simulink model "CCf"  (Simulink 7.5)
settings: Solver=ode45  StartTime=0.0  StopTime=60  RelTol=1e-3
StartFcn:
  | faHPGR=[0.0239 0.4001 0.2089 0.1090 0.0549 0.0441 0.0542 0.0374 0.0159 0.0085 0.0088 0.0085 0.0258]
settings Model: Creator=Fer  LastModifiedBy=Fer

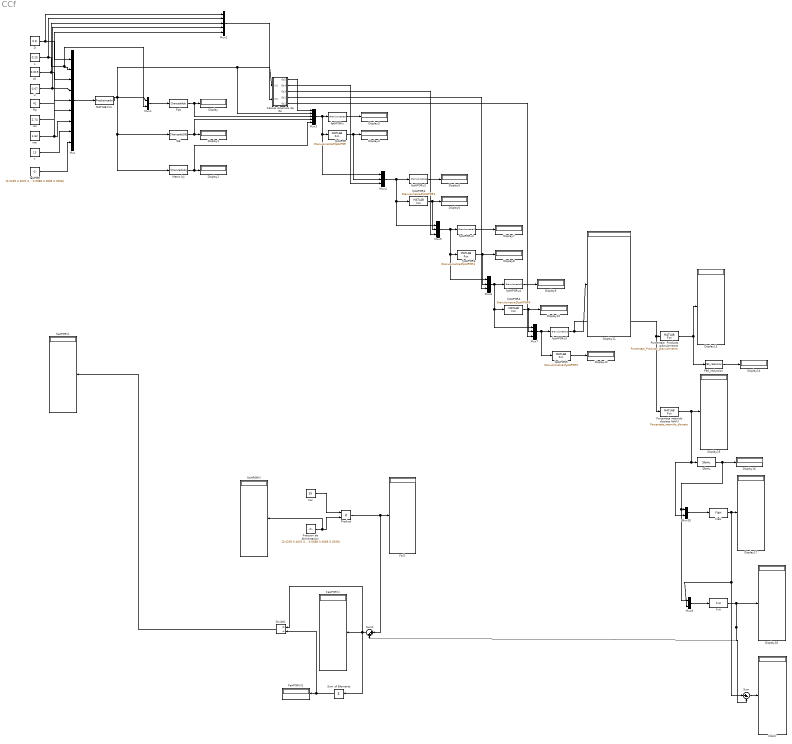
== system CCf ==
  Calculo dinamico de Gs : Subsystem
  D : Constant  Value=0.8  OutDataType=fixdt(1, 16)  OutScaling=2^0
  Display{,1..18} (19 alike) : Display
  Divide1 : Product  Inputs=*/  OutDataType=fixdt(1, 16)  OutScaling=2^-10
  Fa(i) : Display
  FaHPGR(i) : Display
  FaHPGR(i)1 : Display
  Fal : Constant  Value=35  OutDataType=fixdt(1, 16)  OutScaling=2^0
  FdH(i) : Display
  FlaH : MATLABFcn  MATLABFcn=FlaH
  FrH : MATLABFcn  MATLABFcn=FrH
  Fraccion de Alimentacion : Constant  Value=[0.0239 0.4001 0.2089 0.1090 0.0549 0.0441 0.0542 0.0374 0.0159 0.0085 0.0088 0.0085 0.0258]  OutDataType=fixdt(1, 16)  OutScaling=2^0
  L : Constant  Value=0.25  OutDataType=fixdt(1, 16)  OutScaling=2^0
  MATLAB Fcn : MATLABFcn  MATLABFcn=Prechancado
  Matriz bij : MATLABFcn  MATLABFcn=Chancadobij
  Mux : Mux  Inputs=9
  Mux1 : Mux  Inputs=2
  Mux2 : Mux  Inputs=5
  Mux20 : Mux  Inputs=2
  Mux3 : Mux  Inputs=5
  Mux{4..7} (4 alike) : Mux  Inputs=3
  Mux8 : Mux  Inputs=2
  P80_reduccion : MATLABFcn  MATLABFcn=P80_reduccion
  Porcentaje  Producto granulometria : MATLABFcn  MATLABFcn=Porcentaje_Producto_granulometria
  Porcentaje retenido discreto faH(i) : MATLABFcn  MATLABFcn=Porcentaje_retenido_discreto
  Ppb : MATLABFcn  MATLABFcn=ChancadoPpb
  Product : Product  OutDataType=fixdt(1, 16)  OutScaling=2^0  RndMeth=Zero
  Rp : Constant  Value=41  OutDataType=fixdt(1, 16)  OutScaling=2^0
  SfaHu : MATLABFcn  MATLABFcn=SfaHu
  SiE : MATLABFcn  MATLABFcn=ChancadoSiE
  Sum : Sum  Inputs=|+-  OutDataType=fixdt(1, 16)  OutScaling=2^0
  Sum of Elements : Sum  Inputs=+  OutDataType=fixdt(1, 16)  OutScaling=2^-10
  Sum1 : Sum  Inputs=|++  OutDataType=fixdt(1, 16)  OutScaling=2^0
  U : Constant  Value=0.67  OutDataType=fixdt(1, 16)  OutScaling=2^0
  faHPGR : Constant  Value=[0.0239 0.4001 0.2089 0.1090 0.0549 0.0441 0.0542 0.0374 0.0159 0.0085 0.0088 0.0085 0.0258]  OutDataType=fixdt(1, 16)  OutScaling=2^0
  faHPGR(i) : Display
  faiHPGR(i) : Display
  fptHPGR : MATLABFcn  MATLABFcn=Granulometria5fptHPGR
  fptHPGR2 : MATLABFcn  MATLABFcn=Granulometria4fptHPGR2
  fptHPGR3 : MATLABFcn  MATLABFcn=Granulometria3fptHPGR3
  fptHPGR4 : MATLABFcn  MATLABFcn=Granulometria2fptHPGR4
  fptHPGR5 : MATLABFcn  MATLABFcn=Granulometria1fptHPGR5
  fptHPGRu : MATLABFcn  MATLABFcn=Granulometria5
  fptHPGRu2 : MATLABFcn  MATLABFcn=Granulometria4
  fptHPGRu3 : MATLABFcn  MATLABFcn=Granulometria3
  fptHPGRu4 : MATLABFcn  MATLABFcn=Granulometria2
  fptHPGRu5 : MATLABFcn  MATLABFcn=Granulometria1
  n : Constant  Value=13  OutDataType=fixdt(1, 16)  OutScaling=2^0
  roa : Constant  Value=1.62  OutDataType=fixdt(1, 16)  OutScaling=2^0
  ros : Constant  Value=2.74  OutDataType=fixdt(1, 16)  OutScaling=2^0
  s0 : Constant  Value=0.019  OutDataType=fixdt(1, 16)  OutScaling=2^0
  wires:
  D/1 -> Mux/1, Mux2/1
  L/1 -> Mux/2, Mux1/2, Mux2/2
  s0/1 -> Mux/3, Mux2/3
  U/1 -> Mux/4, Mux2/4
  Rp/1 -> Mux/5
  ros/1 -> Mux/6
  roa/1 -> Mux/7, Mux2/5
  n/1 -> Mux/8
  MATLAB Fcn/1 -> Mux1/1, SiE/1, Matriz bij/1, Calculo dinamico de Gs/1(In1), Mux3/2
  Mux/1 -> MATLAB Fcn/1
  Mux1/1 -> Ppb/1
  Ppb/1 -> Display/1, Mux3/3
  SiE/1 -> Display1/1, Mux3/4
  Mux2/1 -> Calculo dinamico de Gs/2(In2)
  Matriz bij/1 -> Display2/1, Mux3/5
  Calculo dinamico de Gs/1(Gs5) -> Mux3/1
  Calculo dinamico de Gs/2(Gs4) -> Mux4/3
  Calculo dinamico de Gs/3(Gs3) -> Mux5/3
  Calculo dinamico de Gs/4(Gs2) -> Mux6/3
  Calculo dinamico de Gs/5(Gs1) -> Mux7/3
  Mux3/1 -> fptHPGRu/1, fptHPGR/1, Mux4/1
  fptHPGR/1 -> Display4/1, Mux4/2
  Mux4/1 -> fptHPGRu2/1, fptHPGR2/1, Mux5/1
  fptHPGR2/1 -> Display6/1, Mux5/2
  Mux5/1 -> fptHPGRu3/1, fptHPGR3/1, Mux6/1
  fptHPGR3/1 -> Display8/1, Mux6/2
  Mux6/1 -> fptHPGRu4/1, fptHPGR4/1, Mux7/1
  fptHPGR4/1 -> Display10/1, Mux7/2
  Mux7/1 -> fptHPGRu5/1, fptHPGR5/1
  fptHPGR5/1 -> Display12/1
  fptHPGRu/1 -> Display3/1
  fptHPGRu2/1 -> Display5/1
  fptHPGRu3/1 -> Display7/1
  fptHPGRu5/1 -> Display11/1, Porcentaje  Producto granulometria/1, Porcentaje retenido discreto faH(i)/1
  fptHPGRu4/1 -> Display9/1
  Porcentaje  Producto granulometria/1 -> Display13/1, P80_reduccion/1
  P80_reduccion/1 -> Display14/1
  Porcentaje retenido discreto faH(i)/1 -> Display15/1, SfaHu/1, Mux20/2
  SfaHu/1 -> Display16/1, Mux20/1, Mux8/1
  Mux20/1 -> FlaH/1
  FlaH/1 -> Display17/1, Mux8/2, Sum/1
  Mux8/1 -> FrH/1
  FrH/1 -> Display18/1, Sum/2, Sum1/2
  Sum/1 -> FdH(i)/1
  Fal/1 -> Product/1
  Fraccion de Alimentacion/1 -> Product/2, faiHPGR(i)/1
  Product/1 -> Fa(i)/1, Sum1/1
  Sum1/1 -> Divide1/1, Sum of Elements/1, FaHPGR(i)/1
  Sum of Elements/1 -> FaHPGR(i)1/1, Divide1/2
  Divide1/1 -> faHPGR(i)/1
  faHPGR/1 -> Mux/9

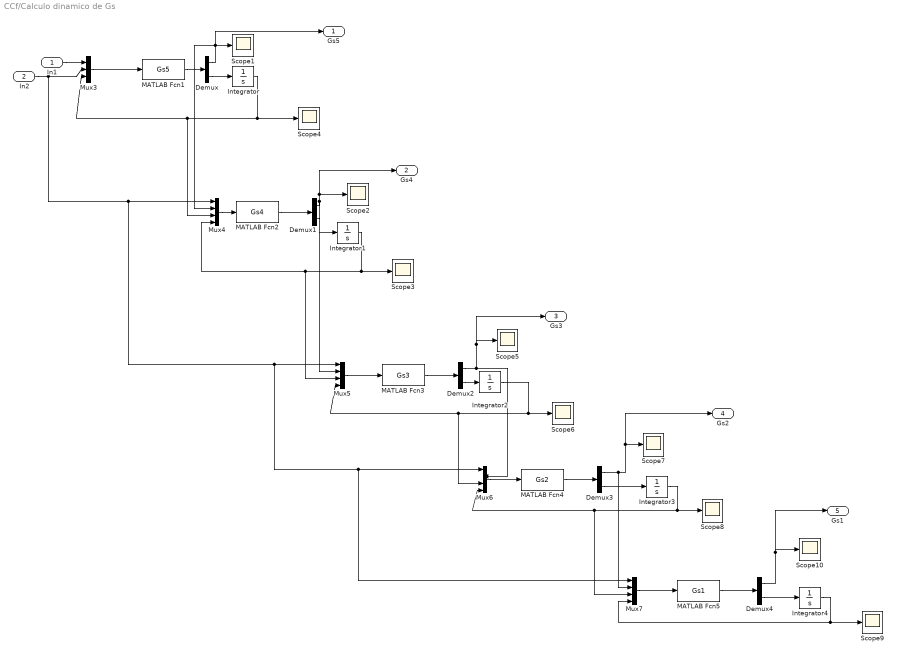
== system CCf/Calculo dinamico de Gs ==
  In1 : Inport
  In2 : Inport  Port=2
  Demux{,1..4} (5 alike) : Demux  Outputs=2
  Integrator{,1..4} (5 alike) : Integrator  InitialCondition=1.6
  MATLAB Fcn1 : MATLABFcn  MATLABFcn=Gs5
  MATLAB Fcn2 : MATLABFcn  MATLABFcn=Gs4
  MATLAB Fcn3 : MATLABFcn  MATLABFcn=Gs3
  MATLAB Fcn4 : MATLABFcn  MATLABFcn=Gs2
  MATLAB Fcn5 : MATLABFcn  MATLABFcn=Gs1
  Mux3 : Mux  Inputs=3
  Mux{4..7} (4 alike) : Mux
  Scope{1..10} (10 alike) : Scope
      Scope10 settings: SaveName=ScopeData9
      Scope3 settings: SaveName=ScopeData2
      Scope4 settings: SaveName=ScopeData3
      Scope5 settings: SaveName=ScopeData4
      Scope6 settings: SaveName=ScopeData5
      Scope7 settings: SaveName=ScopeData6
      Scope8 settings: SaveName=ScopeData7
      Scope9 settings: SaveName=ScopeData8
  Gs5 : Outport  OutDataType=fixdt(1, 16)  OutScaling=2^0
  Gs4 : Outport  Port=2  OutDataType=fixdt(1, 16)  OutScaling=2^0
  Gs3 : Outport  Port=3  OutDataType=fixdt(1, 16)  OutScaling=2^0
  Gs2 : Outport  Port=4  OutDataType=fixdt(1, 16)  OutScaling=2^0
  Gs1 : Outport  Port=5  OutDataType=fixdt(1, 16)  OutScaling=2^0
  wires:
  In2/1 -> Mux7/1, Mux6/1, Mux5/1, Mux4/1, Mux3/2
  Mux3/1 -> MATLAB Fcn1/1
  Integrator/1 -> Mux3/3, Mux4/3, Scope4/1
  MATLAB Fcn1/1 -> Demux/1
  Demux/2 -> Integrator/1
  Demux/1 -> Scope1/1, Mux4/2, Gs5/1
  Integrator1/1 -> Scope3/1, Mux4/4, Mux5/3
  Demux1/2 -> Integrator1/1
  Mux4/1 -> MATLAB Fcn2/1
  MATLAB Fcn2/1 -> Demux1/1
  Demux1/1 -> Mux5/2, Scope2/1, Gs4/1
  Mux5/1 -> MATLAB Fcn3/1
  MATLAB Fcn3/1 -> Demux2/1
  Demux2/2 -> Integrator2/1
  Integrator2/1 -> Scope6/1, Mux5/4, Mux6/3
  Demux2/1 -> Mux6/2, Scope5/1, Gs3/1
  Mux6/1 -> MATLAB Fcn4/1
  MATLAB Fcn4/1 -> Demux3/1
  Demux3/2 -> Integrator3/1
  Integrator3/1 -> Scope8/1, Mux6/4, Mux7/3
  Demux3/1 -> Mux7/2, Scope7/1, Gs2/1
  Mux7/1 -> MATLAB Fcn5/1
  MATLAB Fcn5/1 -> Demux4/1
  Demux4/2 -> Integrator4/1
  Integrator4/1 -> Mux7/4, Scope9/1
  Demux4/1 -> Scope10/1, Gs1/1
  In1/1 -> Mux3/1
